simulink model "ThdRwRtStFwdBkwdEnServer"  (R2018b)
settings: Solver=FixedStepDiscrete  StartTime=0.0  StopTime=10.0  FixedStep=0.01  RelTol=1e-3
libraries: simulink x3
settings Model: Creator=sn2xws  LastModifiedBy=sn2xws
settings DataIOCC: SaveFormat=StructureWithTime
settings OptimizationCC: DefaultParameterBehavior=Inlined  EnhancedBackFolding=on  PassReuseOutputArgsAs=Individual arguments  ZeroExternalMemoryAtStartup=off  ZeroInternalMemoryAtStartup=off  OptimizeBlockOrder=speed  DifferentSizesBufferReuse=on  OptimizationCustomize=off
settings DebuggingCC: ParameterTunabilityLossMsg=error
settings ModelReferenceCC: ModelReferenceNumInstancesAllowed=Single
settings SFSimCC: MATLABDynamicMemAlloc=off
settings RTWCC: SystemTargetFile=autosar.tlc  GenCodeOnly=on  TemplateMakefile=ert_default_tmf  Description=AUTOSAR  GenerateReport=on  IncludeHyperlinkInReport=on  LaunchReport=on  GenerateTraceInfo=on  GenerateTraceReport=on  GenerateTraceReportSl=on  GenerateTraceReportSf=on  GenerateTraceReportEml=on
settings CodeAppCC: ForceParamTrailComments=on  IgnoreCustomStorageClasses=off  OperatorAnnotations=on  SimulinkDataObjDesc=on  SFDataObjDesc=on  InsertBlockDesc=on
settings STFCustomTargetCC: TargetLangStandard=C99 (ISO)  MultiwordLength=256  ParMdlRefBuildCompliant=on  CompOptLevelCompliant=on  IncludeMdlTerminateFcn=off  CombineOutputUpdateFcns=on  SuppressErrorStatus=on  ERTCustomFileBanners=on  SupportNonFinite=off  SupportComplex=off  SupportContinuousTime=off  SupportNonInlinedSFcns=off  RemoveResetFunc=on  MATLABClassNameForMDSCustomization=Simulink.SoftwareTarget.ERTCustomization  AutosarCompliant=on  UseToolchainInfoCompliant=on  LookupTableObjectStructAxisOrder=2,1,3,4,...  LUTObjectStructOrderEvenSpacing=Size,Table,Breakpoints  SystemTargetFile=autosar.tlc
settings ERTTargetCC: TargetLangStandard=C99 (ISO)  ConcurrentExecutionCompliant=off  IncludeMdlTerminateFcn=off  SuppressErrorStatus=on  SupportNonFinite=off  SupportComplex=off  ModelStepFunctionPrototypeControlCompliant=off  CPPClassGenCompliant=off  AutosarCompliant=on  LookupTableObjectStructAxisOrder=2,1,3,4,...  LUTObjectStructOrderEvenSpacing=Size,Table,Breakpoints  InlinedParameterPlacement=NonHierarchical  ERTCustomFileTemplate=example_file_process.tlc  ERTFilePackagingFormat=Compact

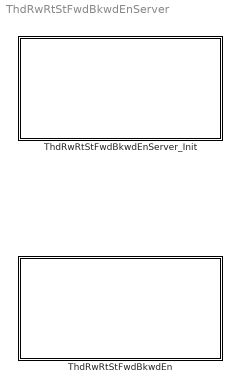
== system ThdRwRtStFwdBkwdEnServer ==
  ThdRwRtStFwdBkwdEn : Subsystem
  ThdRwRtStFwdBkwdEnServer_Init : Subsystem

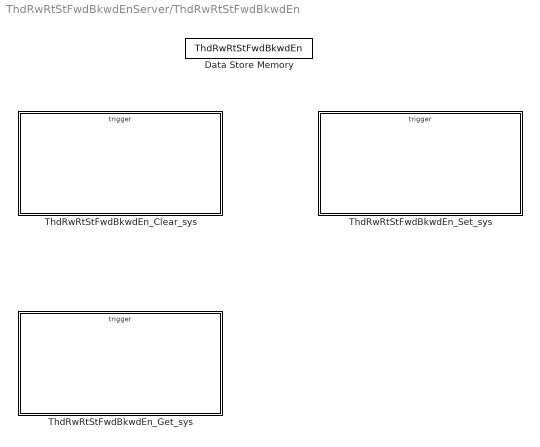
== system ThdRwRtStFwdBkwdEnServer/ThdRwRtStFwdBkwdEn ==
  Data Store Memory : DataStoreMemory  DataStoreName=ThdRwRtStFwdBkwdEn  ReadBeforeWriteMsg=warning  WriteAfterWriteMsg=warning  WriteAfterReadMsg=warning  ShowAdditionalParam=off
      settings: RTWStateStorageClass=ExportedGlobal
  ThdRwRtStFwdBkwdEn_Clear_sys : Subsystem
  ThdRwRtStFwdBkwdEn_Get_sys : Subsystem
  ThdRwRtStFwdBkwdEn_Set_sys : Subsystem

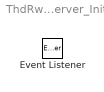
== system ThdRwRtStFwdBkwdEnServer/ThdRwRtStFwdBkwdEnServer_Init ==
  Event Listener : EventListener  EventName=reset

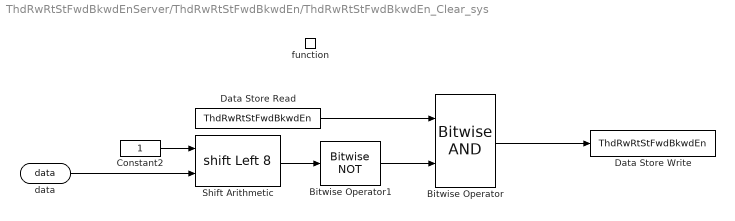
== system ThdRwRtStFwdBkwdEnServer/ThdRwRtStFwdBkwdEn/ThdRwRtStFwdBkwdEn_Clear_sys ==
  function : TriggerPort  TriggerType=function-call  IsSimulinkFunction=on  FunctionName=ThdRwRtStFwdBkwdEn_Clear  VariantControl=(inherit)
  Bitwise Operator : simulink/Logic and Bit Operations/Bitwise Operator  logicop=AND  UseBitMask=off  NumInputPorts=2  BitMask=bin2dec('11011001')  BitMaskRealWorld=Stored Integer
  Bitwise Operator1 : simulink/Logic and Bit Operations/Bitwise Operator  logicop=NOT  UseBitMask=off  BitMask=bin2dec('11011001')  BitMaskRealWorld=Stored Integer
  Constant2 : Constant  OutDataTypeStr=uint32
  Data Store Read : DataStoreRead  DataStoreName=ThdRwRtStFwdBkwdEn
  Data Store Write : DataStoreWrite  DataStoreName=ThdRwRtStFwdBkwdEn
  Shift Arithmetic : ArithShift  BitShiftNumberSource=Input port  BitShiftNumber=8  BitShiftDirection=Left
      settings: InputPortMap=u0,p1
  data : ArgIn  OutDataTypeStr=uint8  ArgumentName=data
  wires:
  Constant2/1 -> Shift Arithmetic/1
  Data Store Read/1 -> Bitwise Operator/1
  Bitwise Operator/1 -> Data Store Write/1
  Shift Arithmetic/1 -> Bitwise Operator1/1
  Bitwise Operator1/1 -> Bitwise Operator/2
  data/1 -> Shift Arithmetic/2

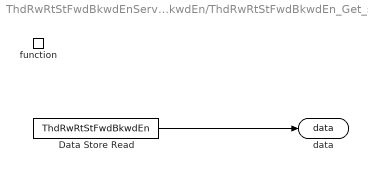
== system ThdRwRtStFwdBkwdEnServer/ThdRwRtStFwdBkwdEn/ThdRwRtStFwdBkwdEn_Get_sys ==
  function : TriggerPort  TriggerType=function-call  IsSimulinkFunction=on  FunctionName=ThdRwRtStFwdBkwdEn_Get  VariantControl=(inherit)
  Data Store Read : DataStoreRead  DataStoreName=ThdRwRtStFwdBkwdEn
  data : ArgOut  OutDataTypeStr=uint32  ArgumentName=data
  wires:
  Data Store Read/1 -> data/1

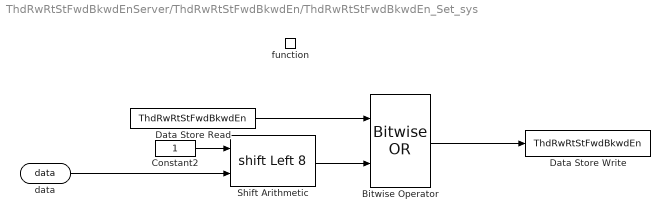
== system ThdRwRtStFwdBkwdEnServer/ThdRwRtStFwdBkwdEn/ThdRwRtStFwdBkwdEn_Set_sys ==
  function : TriggerPort  TriggerType=function-call  IsSimulinkFunction=on  FunctionName=ThdRwRtStFwdBkwdEn_Set  VariantControl=(inherit)
  Bitwise Operator : simulink/Logic and Bit Operations/Bitwise Operator  logicop=OR  UseBitMask=off  NumInputPorts=2  BitMask=bin2dec('11011001')  BitMaskRealWorld=Stored Integer
  Constant2 : Constant  OutDataTypeStr=uint32
  Data Store Read : DataStoreRead  DataStoreName=ThdRwRtStFwdBkwdEn
  Data Store Write : DataStoreWrite  DataStoreName=ThdRwRtStFwdBkwdEn
  Shift Arithmetic : ArithShift  BitShiftNumberSource=Input port  BitShiftNumber=8  BitShiftDirection=Left
      settings: InputPortMap=u0,p1
  data : ArgIn  OutDataTypeStr=uint8  ArgumentName=data
  wires:
  Data Store Read/1 -> Bitwise Operator/1
  Constant2/1 -> Shift Arithmetic/1
  Bitwise Operator/1 -> Data Store Write/1
  Shift Arithmetic/1 -> Bitwise Operator/2
  data/1 -> Shift Arithmetic/2
